simulink model "lqr_design"  (R2025a)
settings: Solver=VariableStepAuto  StartTime=0.0  StopTime=25  RelTol=1e-3
settings Model: Creator=mdnazmusshakib  LastModifiedBy=mdnazmusshakib

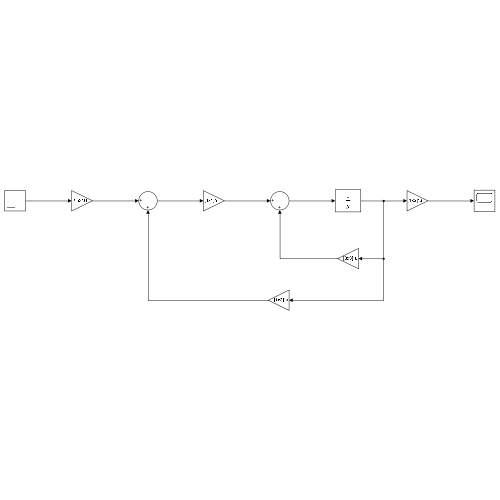
[thumbnail: Simulink's stored preview of the top-level diagram]
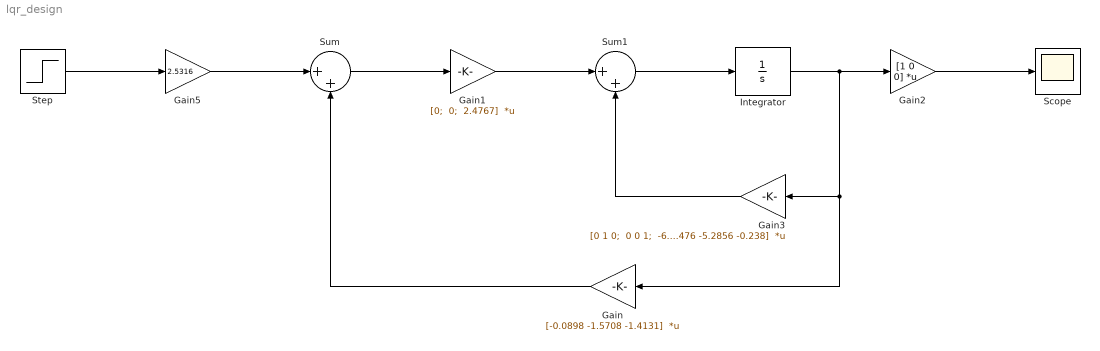
== system lqr_design ==
  Gain : Gain  Gain=[-0.0898 -1.5708 -1.4131]  Multiplication=Matrix(K*u)
  Gain1 : Gain  Gain=|  Multiplication=Matrix(K*u)
      | [0;
      |  0;
      |  2.4767]
  Gain2 : Gain  Gain=[1 0 0]  Multiplication=Matrix(K*u)
  Gain3 : Gain  Gain=|  Multiplication=Matrix(K*u)
      | [0 1 0;
      |  0 0 1;
      |  -6.0476 -5.2856 -0.238]
  Gain5 : Gain  Gain=2.5316
  Integrator : Integrator  InitialCondition=[0; 0; 0]
  Scope : Scope
      settings: ActiveDisplayYMinimum=-3.1250030123971979  ActiveDisplayYMaximum=28.125027111574788
  Step : Step  Time=0  After=16.67  SampleTime=0
  Sum : Sum  Inputs=|++
  Sum1 : Sum  Inputs=|++
  wires:
  Gain1/1 -> Sum1/1
  Sum1/1 -> Integrator/1
  Integrator/1 -> Gain/1, Gain3/1, Gain2/1
  Gain2/1 -> Scope/1
  Gain3/1 -> Sum1/2
  Gain/1 -> Sum/2
  Gain5/1 -> Sum/1
  Sum/1 -> Gain1/1
  Step/1 -> Gain5/1
